simulink model "Controller"  (R2021b)
settings: Solver=VariableStepAuto  StartTime=0.0  StopTime=4  RelTol=1e-3
settings Model: Creator=Fassi  LastModifiedBy=Fassi

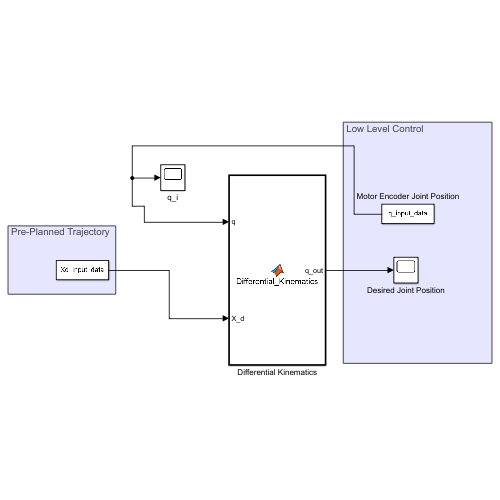
[thumbnail: Simulink's stored preview of the top-level diagram]
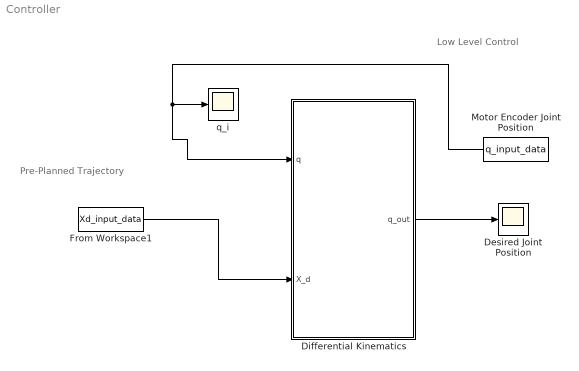
== system Controller ==
  note: Pre-Planned Trajectory
  note: Low Level Control
  Desired Joint Position : Scope
  Differential Kinematics : MATLAB Function  TreatAsAtomicUnit=on
  From Workspace1 : FromWorkspace  VariableName=Xd_input_data  SampleTime=0.01  Interpolate=off  ZeroCross=off  OutputAfterFinalValue=Setting to zero
  Motor Encoder Joint Position : FromWorkspace  VariableName=q_input_data  SampleTime=0.01  Interpolate=off  ZeroCross=off  OutputAfterFinalValue=Setting to zero
  q_i : Scope
  wires:
  Differential Kinematics/1(q_out) -> Desired Joint Position/1
  From Workspace1/1 -> Differential Kinematics/2(X_d)
  Motor Encoder Joint Position/1 -> Differential Kinematics/1(q), q_i/1

== matlab function Controller/Differential Kinematics ==
  data: q input; X_d input; q_out output
function q_out  = Differential_Kinematics(q, X_d)
% Calculates a statistical mean and a standard
% deviation for the values in vals.

l1 = 0.6;
l2 = 0.6;


J = [- l2*sin(q(1) + q(2))-l1*sin(q(1)), -l2*sin(q(1) + q(2)), 0; 
    l2*cos(q(1) + q(2)) + l1*cos(q(1)), l2*cos(q(1) + q(2)), 0
    1,1,1 ];
    if det(J) ~= 0
        delta_q = J\(X_d-ef_pos_from_q(q(1), q(2), q(3), l1, l2));
        q_out = q + delta_q;
    else
        q_out = q;
    end

end


function X = ef_pos_from_q(q1, q2, q3, l1, l2)
%X = [x y phi]
X = [l2*cos(q1 + q2) + l1*cos(q1) l2*sin(q1 + q2) + l1*sin(q1) q1 + q2 + q3]';
end
